simulink model "Controladores"  (R2023b)
settings: Solver=ode4  StartTime=0.0  StopTime=10.0  FixedStep=0.001  RelTol=1e-3
undefined symbols (not defined in the file or in its folder): K, Ki
settings Model: Creator=carlo  LastModifiedBy=carlo

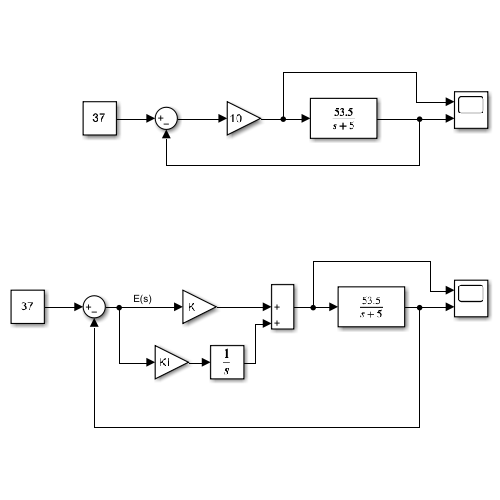
[thumbnail: Simulink's stored preview of the top-level diagram]
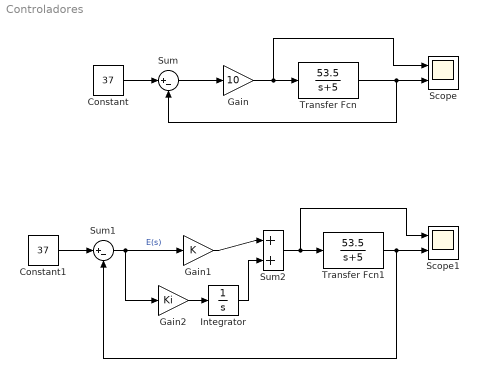
== system Controladores ==
  Constant : Constant  Value=37
  Constant1 : Constant  Value=37
  Gain : Gain  Gain=10
  Gain1 : Gain  Gain=K
  Gain2 : Gain  Gain=Ki
  Integrator : Integrator
  Scope : Scope  NumInputPorts=2
  Scope1 : Scope  NumInputPorts=2
  Sum : Sum  Inputs=|+-
  Sum1 : Sum  Inputs=|+-
  Sum2 : Sum  Inputs=|++
  Transfer Fcn : TransferFcn  Numerator=[53.5]  Denominator=[1 5]
  Transfer Fcn1 : TransferFcn  Numerator=[53.5]  Denominator=[1 5]
  wires:
  Transfer Fcn/1 -> Sum/2, Scope/2
  Gain/1 -> Scope/1, Transfer Fcn/1
  Constant/1 -> Sum/1
  Sum/1 -> Gain/1
  Sum1/1 -> Gain2/1, Gain1/1  "E(s)"
  Constant1/1 -> Sum1/1
  Transfer Fcn1/1 -> Sum1/2, Scope1/2
  Gain1/1 -> Sum2/1
  Sum2/1 -> Scope1/1, Transfer Fcn1/1
  Gain2/1 -> Integrator/1
  Integrator/1 -> Sum2/2
